simulink model "HW9_"  (R2020b)
settings: Solver=VariableStepAuto  StartTime=0.0  StopTime=10.0  RelTol=1e-3
settings Model: Creator=ricky  LastModifiedBy=ricky

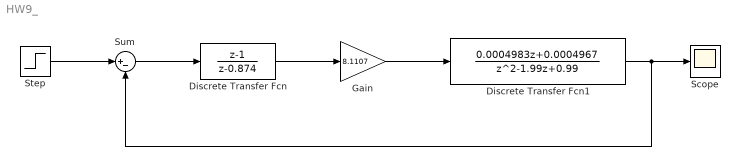
== system HW9_ ==
  Discrete Transfer Fcn : DiscreteTransferFcn  Numerator=[1 -1]  Denominator=[1 -0.874]  SampleTime=0.1
  Discrete Transfer Fcn1 : DiscreteTransferFcn  Numerator=[0.0004983 0.0004967]  Denominator=[1 -1.99 0.99]  SampleTime=0.1
  Gain : Gain  Gain=8.1107
  Scope : Scope
  Step : Step  Time=0  SampleTime=0
  Sum : Sum  Inputs=|+-
  wires:
  Discrete Transfer Fcn/1 -> Gain/1
  Sum/1 -> Discrete Transfer Fcn/1
  Discrete Transfer Fcn1/1 -> Sum/2, Scope/1
  Step/1 -> Sum/1
  Gain/1 -> Discrete Transfer Fcn1/1
